simulink model "scheme"  (R2023b)
settings: Solver=FixedStepAuto  StartTime=0.0  StopTime=1  FixedStep=0.001  MaxStep=0.001  RelTol=1e-3
settings Model: Creator=Катя  LastModifiedBy=Катя

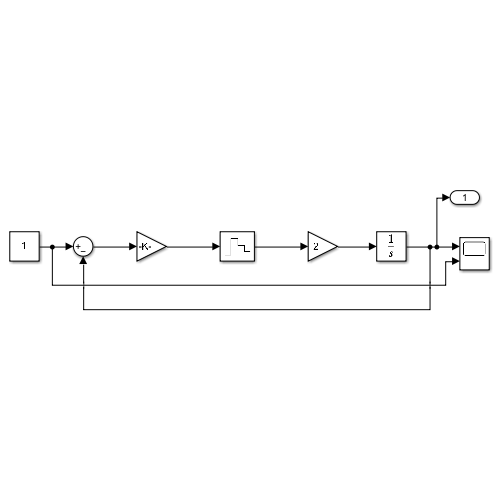
[thumbnail: Simulink's stored preview of the top-level diagram]
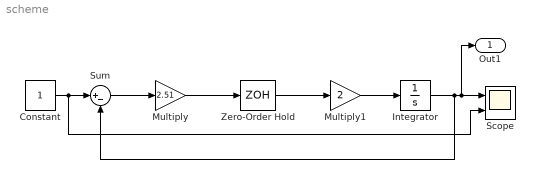
== system scheme ==
  Constant : Constant
  Integrator : Integrator
  Multiply : Gain  Gain=2.51
  Multiply1 : Gain  Gain=2
  Scope : Scope  NumInputPorts=2
  Sum : Sum  Inputs=|+-
  Zero-Order Hold : ZeroOrderHold  SampleTime=0.2
  Out1 : Outport
  wires:
  Sum/1 -> Multiply/1
  Multiply/1 -> Zero-Order Hold/1
  Multiply1/1 -> Integrator/1
  Integrator/1 -> Out1/1, Scope/1, Sum/2
  Zero-Order Hold/1 -> Multiply1/1
  Constant/1 -> Scope/2, Sum/1
